simulink subsystem "PID_AW"  (R2020a)
settings: Solver=VariableStepAuto  StartTime=0.0  StopTime=10.0  RelTol=1e-3
values from neighbouring files (symbols this model uses):
  h_bar = 90    [lab7.mat]
  K_c = 2.0389    [lab7.mat]
  K_i = 0.1887    [lab7.mat]
  u_bar =     [lab7.mat]
settings Model: Creator=bruno  LastModifiedBy=bruno

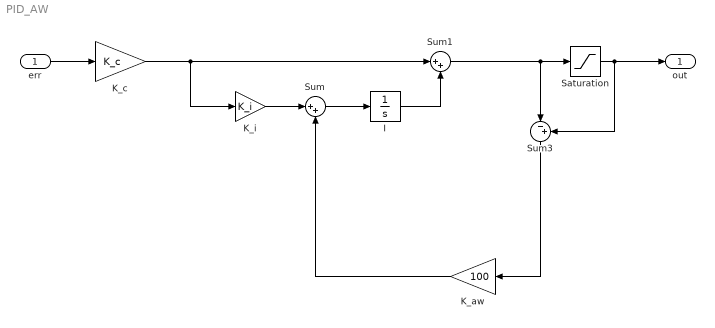
== system PID_AW ==
  err : Inport
  I : Integrator
  K_aw : Gain  Gain=100
  K_c : Gain  Gain=K_c
  K_i : Gain  Gain=K_i
  Saturation : Saturate  UpperLimit=100 - 0.001 - u_bar(h_bar)  LowerLimit=0.001 - u_bar(h_bar)
  Sum : Sum  Inputs=|++
  Sum1 : Sum  Inputs=|++
  Sum3 : Sum  Inputs=|-+
  out : Outport
  wires:
  I/1 -> Sum1/2
  Sum1/1 -> Sum3/1, Saturation/1
  Saturation/1 -> out/1, Sum3/2
  K_c/1 -> Sum1/1, K_i/1
  Sum3/1 -> K_aw/1
  err/1 -> K_c/1
  K_aw/1 -> Sum/2
  Sum/1 -> I/1
  K_i/1 -> Sum/1
